simulink model "msubsys_convert"  (Simulink 7.6)
settings: Solver=ode45  StartTime=0.0  StopTime=10.0  RelTol=1e-3
settings Model: Creator=mtocci  LastModifiedBy=mtocci

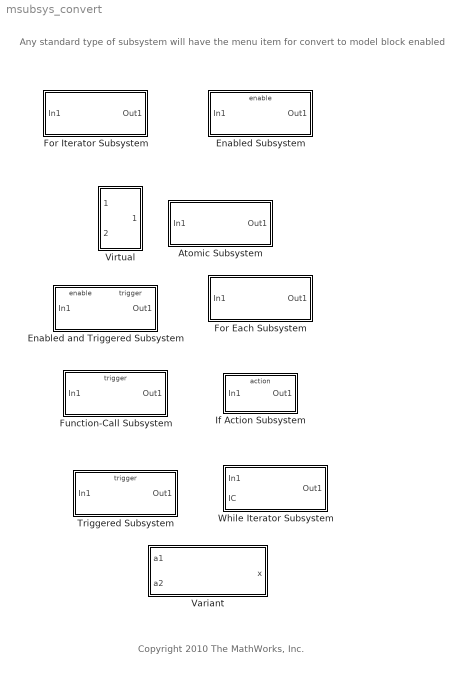
== system msubsys_convert ==
  note: Any standard type of subsystem will
      | have the menu item for convert to model block enabled
  note: Copyright 2010 The MathWorks, Inc.
  Atomic Subsystem : Subsystem  TreatAsAtomicUnit=on
  Enabled Subsystem : Subsystem  TreatAsAtomicUnit=on
  Enabled and Triggered Subsystem : Subsystem  TreatAsAtomicUnit=on
  For Each Subsystem : Subsystem  TreatAsAtomicUnit=on
  For Iterator Subsystem : Subsystem  TreatAsAtomicUnit=on
  Function-Call Subsystem : Subsystem  TreatAsAtomicUnit=on
  If Action Subsystem : Subsystem  TreatAsAtomicUnit=on
  Triggered Subsystem : Subsystem  TreatAsAtomicUnit=on
  Variant : Subsystem  Variant=on
  Virtual : Subsystem
  While Iterator Subsystem : Subsystem  TreatAsAtomicUnit=on

== system msubsys_convert/Atomic Subsystem ==
  In1 : Inport
  Out1 : Outport
  wires:
  In1/1 -> Out1/1

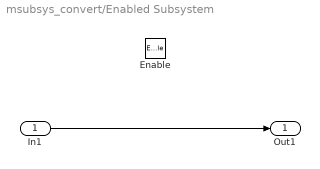
== system msubsys_convert/Enabled Subsystem ==
  In1 : Inport
  Enable : EnablePort
  Out1 : Outport
  wires:
  In1/1 -> Out1/1

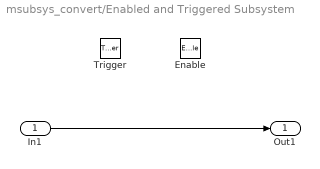
== system msubsys_convert/Enabled and Triggered Subsystem ==
  In1 : Inport
  Enable : EnablePort
  Trigger : TriggerPort
  Out1 : Outport
  wires:
  In1/1 -> Out1/1

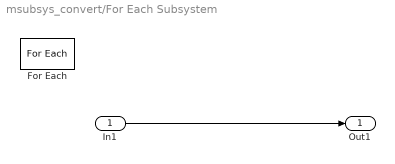
== system msubsys_convert/For Each Subsystem ==
  In1 : Inport  Partition=on  PartitionDimension=1  PartitionWidth=1
  For Each : ForEach  DisableCoverage=on  IndexMode=One-based
  Out1 : Outport  ConcatenationDimension=1
  wires:
  In1/1 -> Out1/1

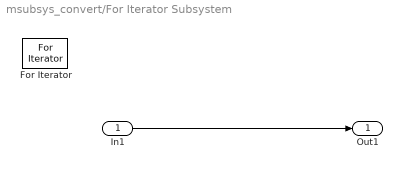
== system msubsys_convert/For Iterator Subsystem ==
  In1 : Inport
  For Iterator : ForIterator
  Out1 : Outport
  wires:
  In1/1 -> Out1/1

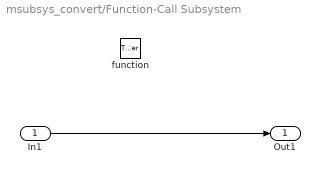
== system msubsys_convert/Function-Call Subsystem ==
  In1 : Inport
  function : TriggerPort  TriggerType=function-call
  Out1 : Outport
  wires:
  In1/1 -> Out1/1

== system msubsys_convert/If Action Subsystem ==
  In1 : Inport
  Action Port : ActionPort
  Out1 : Outport
  wires:
  In1/1 -> Out1/1

== system msubsys_convert/Triggered Subsystem ==
  In1 : Inport
  Trigger : TriggerPort
  Out1 : Outport
  wires:
  In1/1 -> Out1/1

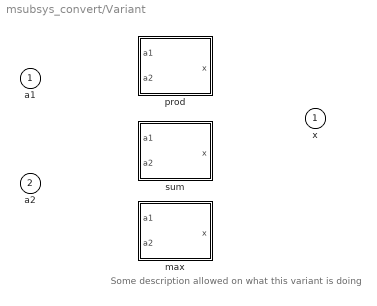
== system msubsys_convert/Variant ==
  note: Some description allowed on what this variant is doing
  a1 : Inport
  a2 : Inport  Port=2
  max : Subsystem  VariantObject=varMax
  prod : Subsystem  VariantObject=varProd
  sum : Subsystem  VariantObject=varSum
  x : Outport  InitialOutput=0

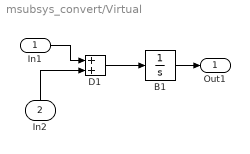
== system msubsys_convert/Virtual ==
  In1 : Inport
  In2 : Inport  Port=2
  B1 : Integrator
  D1 : Sum  SaturateOnIntegerOverflow=on  InputSameDT=on  OutDataTypeStr=Inherit: Same as first input
  Out1 : Outport
  wires:
  D1/1 -> B1/1
  In2/1 -> D1/2
  B1/1 -> Out1/1
  In1/1 -> D1/1

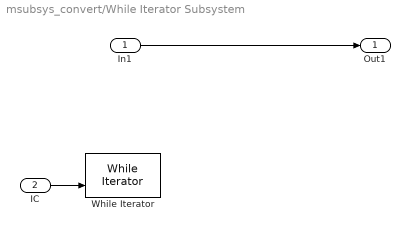
== system msubsys_convert/While Iterator Subsystem ==
  In1 : Inport
  IC : Inport  Port=2
  While Iterator : WhileIterator
  Out1 : Outport
  wires:
  IC/1 -> While Iterator/2
  In1/1 -> Out1/1

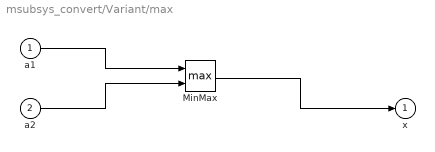
== system msubsys_convert/Variant/max ==
  a1 : Inport
  a2 : Inport  Port=2
  MinMax : MinMax  Function=max  Inputs=2
  x : Outport  InitialOutput=0
  wires:
  MinMax/1 -> x/1
  a2/1 -> MinMax/2
  a1/1 -> MinMax/1

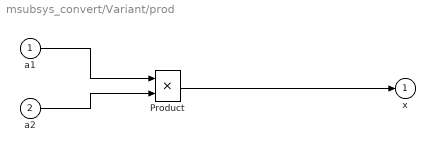
== system msubsys_convert/Variant/prod ==
  a1 : Inport
  a2 : Inport  Port=2
  Product : Product  SaturateOnIntegerOverflow=on  RndMeth=Zero  InputSameDT=on  OutDataTypeStr=Inherit: Same as first input
  x : Outport  InitialOutput=0
  wires:
  a2/1 -> Product/2
  a1/1 -> Product/1
  Product/1 -> x/1

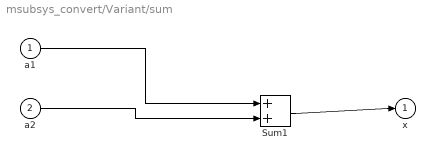
== system msubsys_convert/Variant/sum ==
  a1 : Inport
  a2 : Inport  Port=2
  Sum1 : Sum  SaturateOnIntegerOverflow=on  InputSameDT=on  OutDataTypeStr=Inherit: Same as first input
  x : Outport  InitialOutput=0
  wires:
  a2/1 -> Sum1/2
  a1/1 -> Sum1/1
  Sum1/1 -> x/1
